simulink model "Q5_sim"  (R2022b)
settings: Solver=VariableStepAuto  StartTime=0.0  StopTime=20  RelTol=1e-3
settings Model: Creator=beni  LastModifiedBy=beni

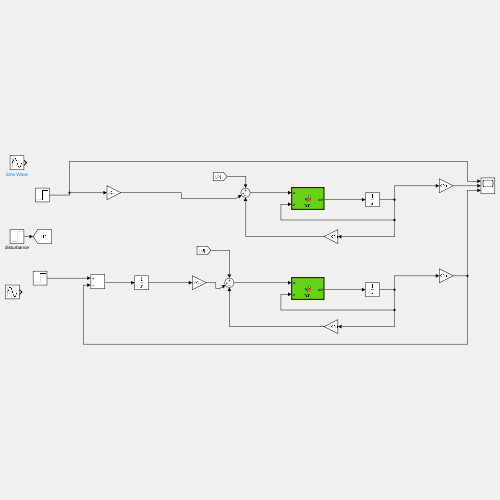
[thumbnail: Simulink's stored preview of the top-level diagram]
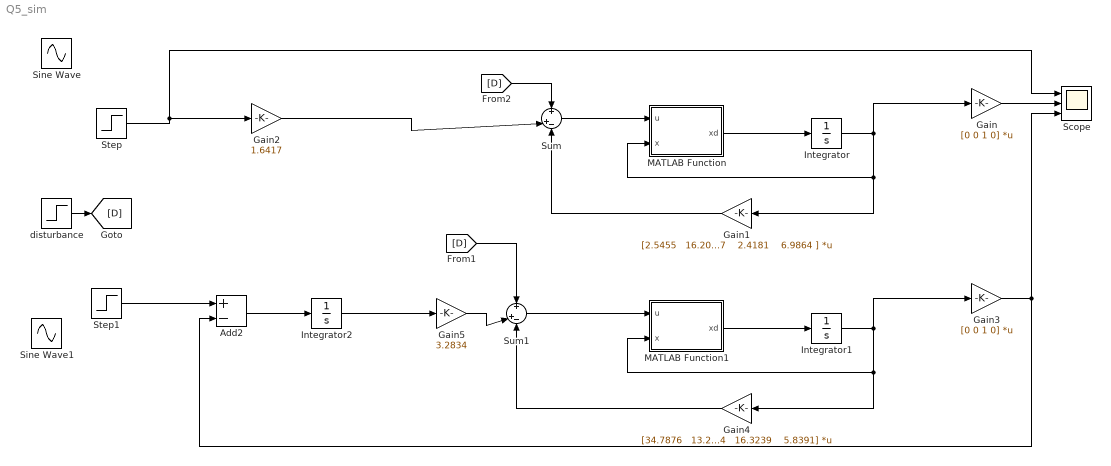
== system Q5_sim ==
  Add2 : Sum  Inputs=+-
  Gain : Gain  Gain=[0 0 1 0]  Multiplication=Matrix(K*u)
  Gain1 : Gain  Gain=|  Multiplication=Matrix(K*u)
      | [2.5455   16.2067    2.4181    6.9864
      | ]
  Gain2 : Gain  Gain=1.6417
  Gain3 : Gain  Gain=[0 0 1 0]  Multiplication=Matrix(K*u)
  Gain4 : Gain  Gain="[34.7876   13.2984   16.3239    5.8391]"  Multiplication=Matrix(K*u)
  Gain5 : Gain  Gain=3.2834
  Integrator : Integrator  InitialCondition=[0;0;0;0]
  Integrator1 : Integrator  InitialCondition=[0;0;0;0]
  Integrator2 : Integrator
  MATLAB Function : MATLAB Function  TreatAsAtomicUnit=on
  MATLAB Function1 : MATLAB Function  TreatAsAtomicUnit=on
  Scope : Scope  NumInputPorts=3
  Sine Wave : Sin  Amplitude=0.1  Frequency=0.5  SampleTime=0
  Sine Wave1 : Sin  SampleTime=0
  Step : Step  After=3.14  SampleTime=0
  Step1 : Step  After=3.14  SampleTime=0
  Sum : Sum  Inputs=+|+-
  Sum1 : Sum  Inputs=+|+-
  disturbance : Step  Time=7  SampleTime=0
  wires:
  MATLAB Function/1(xd) -> Integrator/1
  Integrator/1 -> MATLAB Function/2(x), Gain1/1, Gain/1
  Gain/1 -> Scope/2
  Step/1 -> Gain2/1, Scope/1
  MATLAB Function1/1(xd) -> Integrator1/1
  Integrator1/1 -> Gain4/1, MATLAB Function1/2(x), Gain3/1
  Gain3/1 -> Add2/2, Scope/3
  Step1/1 -> Add2/1
  Add2/1 -> Integrator2/1
  Integrator2/1 -> Gain5/1
  Sum/1 -> MATLAB Function/1(u)
  Sum1/1 -> MATLAB Function1/1(u)
  disturbance/1 -> [D]
  [D] -> Sum1/1
  Gain4/1 -> Sum1/3
  Gain5/1 -> Sum1/2
  Gain1/1 -> Sum/3
  Gain2/1 -> Sum/2
  [D] -> Sum/1

== matlab function Q5_sim/MATLAB Function ==
  data: u input; xd output; x input
function xd= fcn(u,x)

A1 =[0    1.0000         0         0;
   -1.7560   -0.0591    0.0109    0.0005;
         0         0         0    1.0000;
    0.0139    0.0005   -1.3810   -0.0595];

B1=[0;
  -16.0100;
         0;
   38.8400];

xd = A1*x+B1*u;

== matlab function Q5_sim/MATLAB Function1 ==
  data: u input; xd output; x input
function xd= fcn(u,x)

A1 =[0    1.0000         0         0;
   -1.7560   -0.0591    0.0109    0.0005;
         0         0         0    1.0000;
    0.0139    0.0005   -1.3810   -0.0595];

B1=[0;
  -16.0100;
         0;
   38.8400];

xd = A1*x+B1*u;
